simulink model "v1_lqr"  (R2023b)
settings: Solver=VariableStepAuto  StartTime=0.0  StopTime=50  RelTol=1e-3
values from neighbouring files (symbols this model uses):
  K = [double(sol.k1) double(sol.k2)]    [WP2.m]    (also in lqr.m = lqr(sys, Qx, Qu))
  u_eq = 1.003    [WP2.m]    (also in lqr.m)
  x_eq = [x1_eq; x2_eq]    [WP2.m]
settings Model: Creator=kiraa  LastModifiedBy=kiraa

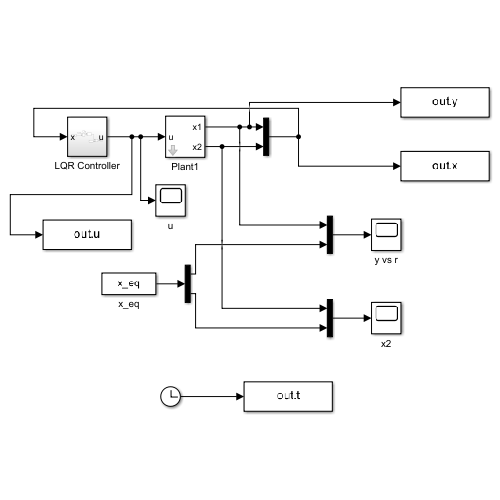
[thumbnail: Simulink's stored preview of the top-level diagram]
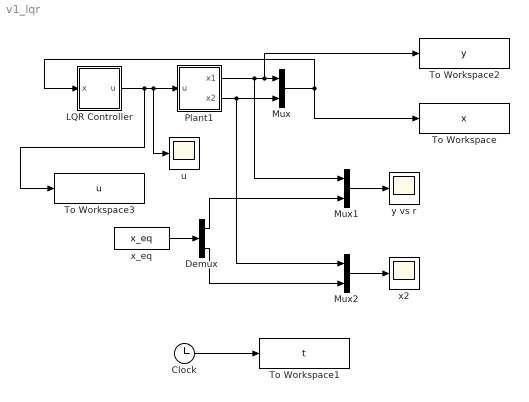
== system v1_lqr ==
  Clock : Clock
  Demux : Demux  Outputs=2
  LQR Controller : Subsystem
  Mux : Mux  Inputs=2
  Mux1 : Mux  Inputs=2
  Mux2 : Mux  Inputs=2
  Plant1 : Subsystem  mask{x1_0=0.7, x2_0=0}
      mask prompts: x1_0 "x1(0) [g/l]"; x2_0 "x2(0) [min^-1]"
  To Workspace : ToWorkspace  VariableName=x  SampleTime=-1
  To Workspace1 : ToWorkspace  VariableName=t  SaveFormat=Timeseries  SampleTime=-1
  To Workspace2 : ToWorkspace  VariableName=y  SampleTime=-1
  To Workspace3 : ToWorkspace  VariableName=u  SampleTime=-1
  u : Scope
  x2 : Scope
  x_eq : Constant  Value=x_eq
  y vs r : Scope
  wires:
  Plant1/2(x2) -> Mux2/1, Mux/2
  Mux/1 -> To Workspace/1, LQR Controller/1(x)
  Mux1/1 -> y vs r/1
  Demux/1 -> Mux1/2
  x_eq/1 -> Demux/1
  Demux/2 -> Mux2/2
  Mux2/1 -> x2/1
  Plant1/1(x1) -> To Workspace2/1, Mux/1, Mux1/1
  Clock/1 -> To Workspace1/1
  LQR Controller/1(u) -> To Workspace3/1, Plant1/1(u), u/1

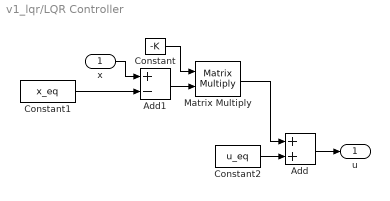
== system v1_lqr/LQR Controller ==
  x : Inport
  Add : Sum
  Add1 : Sum  Inputs=+-  InputSameDT=on  LockScale=on
  Constant : Constant  Value=-K  VectorParams1D=off
  Constant1 : Constant  Value=x_eq
  Constant2 : Constant  Value=u_eq
  Matrix Multiply : Product  Multiplication=Matrix(*)
  u : Outport
  wires:
  Add1/1 -> Matrix Multiply/2
  Constant/1 -> Matrix Multiply/1
  Matrix Multiply/1 -> Add/1
  Add/1 -> u/1
  Constant2/1 -> Add/2
  Constant1/1 -> Add1/2
  x/1 -> Add1/1

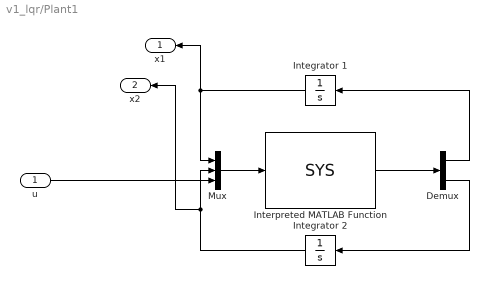
== system v1_lqr/Plant1 ==
  u : Inport
  Demux : Demux  Outputs=2
  Integrator 1 : Integrator  InitialCondition=x1_0
  Integrator 2 : Integrator  InitialCondition=x2_0
  Interpreted MATLAB Function : MATLABFcn  MATLABFcn=SYS  OutputDimensions=2
  Mux : Mux  Inputs=3
  x1 : Outport
  x2 : Outport  Port=2
  wires:
  Integrator 1/1 -> x1/1, Mux/1
  Demux/1 -> Integrator 1/1
  Mux/1 -> Interpreted MATLAB Function/1
  Integrator 2/1 -> x2/1, Mux/2
  Interpreted MATLAB Function/1 -> Demux/1
  Demux/2 -> Integrator 2/1
  u/1 -> Mux/3
